simulink model "sim_assignment_drive"  (R2025b)
settings: Solver=VariableStepAuto  StartTime=0.0  StopTime=5*tau_tes  RelTol=1e-3
values from neighbouring files (symbols this model uses):
  conv = 3/Nav    (= 4.98173364331e-24)    [ass1_fuelcycle_cycle.m]    (also in ass1_steady_state.m)
  Efus_J = Efus*1.602e-13    (= 2.81952e-12)    [ass1_fuelcycle_cycle.m]    (also in ass1_steady_state.m)
  eta_tes = 0.9    [ass1_fuelcycle_cycle.m]    (also in ass1_steady_state.m)
  f_dir = 0.3    [ass1_fuelcycle_cycle.m]    (also in ass1_steady_state.m)
  I_inventory = I_inventory + 50    (= 1450)    [ass1_fuelcycle_cycle.m]    (also in ass1_steady_state.m)
  lambda = 1.83e-9    (= 1.83e-09)    [ass1_fuelcycle_cycle.m]    (also in ass1_steady_state.m)
  Pfus = 500e6    (= 500000000)    [ass1_fuelcycle_cycle.m]    (also in ass1_steady_state.m)
  pulse_width = t_pulse/t_period    (= 0.882352941176)    [ass1_fuelcycle_cycle.m]    (also in ass1_steady_state.m)
  t_period = t_pulse + t_dwell    (= 1020)    [ass1_fuelcycle_cycle.m]    (also in ass1_steady_state.m)
  tau_bb = 3600    [ass1_fuelcycle_cycle.m]    (also in ass1_steady_state.m)
  tau_cp = n_pumps*Mol_H/MolFR_H    [ass1_fuelcycle_cycle.m]    (also in ass1_steady_state.m)
  tau_hx = 3600    [ass1_fuelcycle_cycle.m]    (also in ass1_steady_state.m)
  tau_p = 6*3600    (= 21600)    [ass1_fuelcycle_cycle.m]    (also in ass1_steady_state.m)
  tau_tes = 24*3600    (= 86400)    [ass1_fuelcycle_cycle.m]    (also in ass1_steady_state.m)
  TBE = 0.01    [ass1_fuelcycle_cycle.m]    (also in ass1_steady_state.m)
settings Model: Creator=franc  LastModifiedBy=vairp

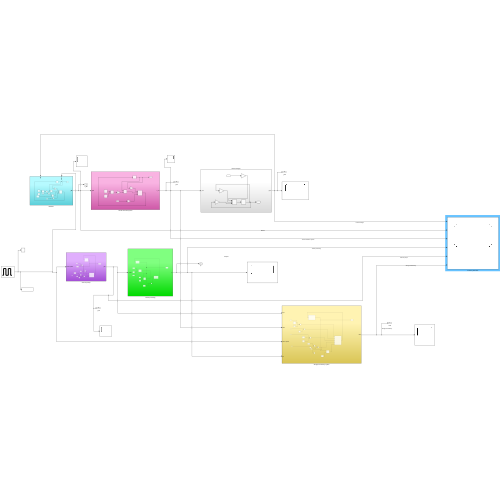
[thumbnail: Simulink's stored preview of the top-level diagram]
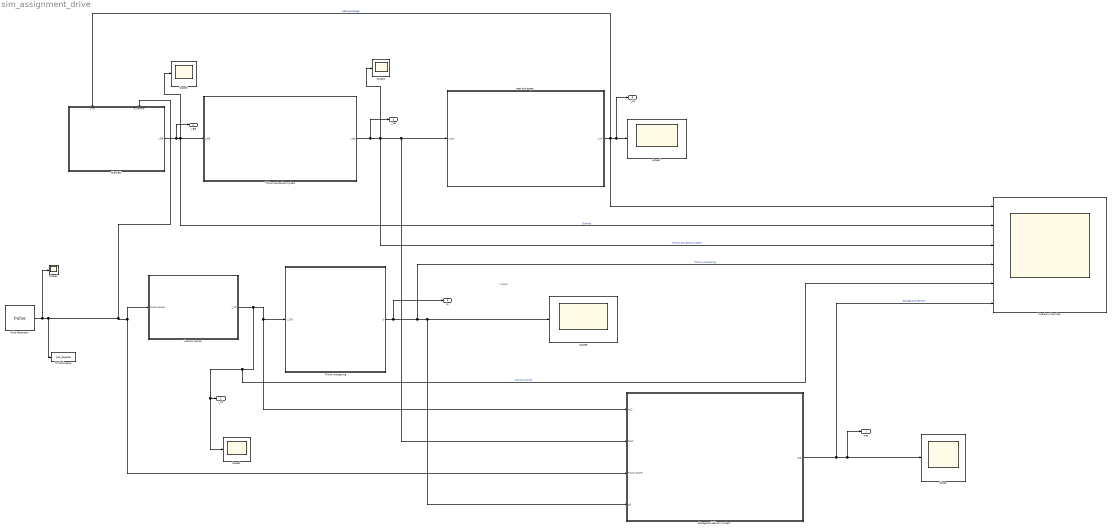
== system sim_assignment_drive ==
  note: scopew
  Blanket1 : Subsystem
      settings: PortSchema="{\"entries\":[{\"content\":{\"sides\":[{\"content\":{},\"type\":\"ConnectorPlacement.EquallySpacedRectSide\",\"uuid\":\"89bca18e-32ff-45a0-b030-61f554edbcca\"},{\"content\":{\"connectorIds\":[\"Out1\"],\"side\":\"RIGHT\"},\"type\":\"ConnectorPlacement.EquallySpacedRectSide\",\"uuid\":\"cf46e808-8a5d-458b-80f9-3800ce8b9836\"},{\"content\":{\"connectorIds\":[\"In1\",\"In2\"],\"side\":\"TOP\"},\"type\":\"ConnectorPlacement.EquallySpacedRectSide\",\"uuid\":\"39017523-1075-4513-926d-a7f0d16af0bc\"},{\"content\":{\"side\":\"BOTTOM\"},\"type\":\"ConnectorPlacement.EquallySpacedRectSide\",\"uuid\":\"04c0dc08-a93f-4928-be32-40ebfd4b2de5\"}]},\"type\":\"ConnectorPlacement.EquallySpacedConnector\",\"uuid\":\"6c4882b1-7a3e-4492-b971-e4bf86d91c33\"}],\"packageUris\":[\"http://schema.mathworks.com/mf0/Connector/R2020b\"],\"version\":\"1.0\"}"
  Heat exchanger : Subsystem
  Inventory Overview : Scope  NumInputPorts=6
      settings: ActiveDisplayYMinimum=-0.43034778362690795  ActiveDisplayYMaximum=3.8731300526421726  YLabel=Trtium inventory [g]  DataLoggingVariableName=ScopeData7
  Pulse Generator : DiscretePulseGenerator  PulseType=Time based  Amplitude=Pfus  Period=t_period  PulseWidth=pulse_width*100
  Scope{,1..5,7} (7 alike) : Scope
      Scope settings: ActiveDisplayYMinimum=35.349526834530543  ActiveDisplayYMaximum=54.275962480479521
      Scope1 settings: ActiveDisplayYMinimum=161.53440000057978  ActiveDisplayYMaximum=182.06300437811379
      Scope2 settings: ActiveDisplayYMinimum=-0.24605784431503164  ActiveDisplayYMaximum=3.8524924759412356  DataLoggingVariableName=ScopeData2
      Scope3 settings: ActiveDisplayYMinimum=-10.069495783527454  ActiveDisplayYMaximum=90.6254620517471  DataLoggingVariableName=ScopeData3
      Scope4 settings: ActiveDisplayYMinimum=-3.526352901457572E+7  ActiveDisplayYMaximum=5.0463497006759679E+8  DataLoggingVariableName=ScopeData4
      Scope5 settings: ActiveDisplayYMinimum=1163.0001078029038  ActiveDisplayYMaximum=1167.301162663447  DataLoggingVariableName=ScopeData5
      Scope7 settings: ActiveDisplayYMinimum=0.33167850023106693  ActiveDisplayYMaximum=0.33586626341534481  DataLoggingVariableName=ScopeData8
  Storage and delivery system : Subsystem
  To Workspace : ToWorkspace  VariableName=out_square  SaveFormat=Timeseries  SampleTime=-1
  Tritium extraction system : Subsystem
  Tritium processing : Subsystem
  Vacuum pumps : Subsystem
  Isds : Outport
  I_CP : Outport  Port=2
  Ip : Outport  Port=3
  I_BB : Outport  Port=4
  I_tes : Outport  Port=5
  I_HX : Outport  Port=6
  wires:
  Pulse Generator/1 -> Scope4/1, To Workspace/1, Storage and delivery system/3(Fusion power), Vacuum pumps/1(Fusion power), Blanket1/2(P_fusione)
  Vacuum pumps/1(I_CP) -> Inventory Overview/5, Scope1/1, I_CP/1, Storage and delivery system/1(Icp2), Tritium processing/1(I_CP2)  "Vacuum pumps"
  Heat exchanger/1(I_HX) -> I_HX/1, Scope7/1, Blanket1/1(I_HX), Inventory Overview/1  "Heat exchanger"
  Blanket1/1(I_BB) -> I_BB/1, Inventory Overview/2, Scope2/1, Tritium extraction system/1(I_BB)  "Blanket"
  Tritium extraction system/1(I_tes) -> I_tes/1, Inventory Overview/3, Scope3/1, Storage and delivery system/2(Ites2), Heat exchanger/1(I_tes)  "Tritium extraction system"
  Storage and delivery system/1(Isds) -> Inventory Overview/6, Isds/1, Scope/1  "Storage and delivery"
  Tritium processing/1(Ip) -> Ip/1, Inventory Overview/4, Storage and delivery system/4(Ip3), Scope5/1  "Tritium processing"

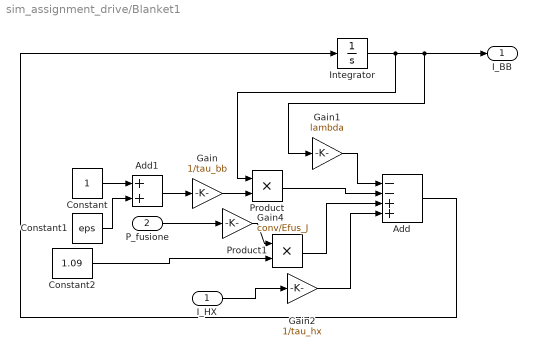
== system sim_assignment_drive/Blanket1 ==
  I_HX : Inport
  P_fusione : Inport  Port=2
  Add : Sum  Inputs=--++
  Add1 : Sum
  Constant : Constant
  Constant1 : Constant  Value=eps
  Constant2 : Constant  Value=1.09
  Gain : Gain  Gain=1/tau_bb
  Gain1 : Gain  Gain=lambda
  Gain2 : Gain  Gain=1/tau_hx
  Gain4 : Gain  Gain=conv/Efus_J
  Integrator : Integrator
  Product : Product
  Product1 : Product
  I_BB : Outport
  wires:
  Product1/1 -> Add/3
  Gain2/1 -> Add/4
  I_HX/1 -> Gain2/1
  Gain1/1 -> Add/1
  Product/1 -> Add/2
  Integrator/1 -> I_BB/1, Gain1/1, Product/1
  Gain/1 -> Product/2
  Add1/1 -> Gain/1
  Constant/1 -> Add1/1
  Constant1/1 -> Add1/2
  Add/1 -> Integrator/1
  Gain4/1 -> Product1/1
  Constant2/1 -> Product1/2
  P_fusione/1 -> Gain4/1

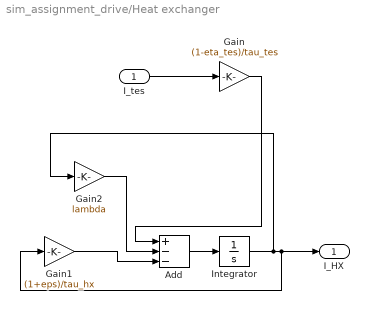
== system sim_assignment_drive/Heat exchanger ==
  I_tes : Inport
  Add : Sum  Inputs=+--
  Gain : Gain  Gain=(1-eta_tes)/tau_tes
  Gain1 : Gain  Gain=(1+eps)/tau_hx
  Gain2 : Gain  Gain=lambda
  Integrator : Integrator
  I_HX : Outport
  wires:
  I_tes/1 -> Gain/1
  Integrator/1 -> Gain2/1, Gain1/1, I_HX/1
  Gain/1 -> Add/1
  Gain1/1 -> Add/3
  Gain2/1 -> Add/2
  Add/1 -> Integrator/1

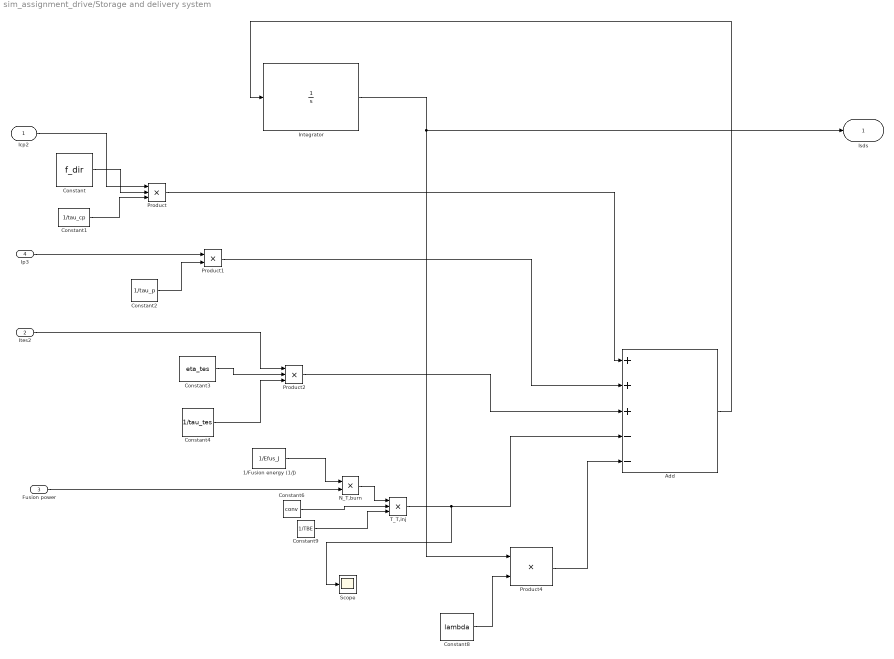
== system sim_assignment_drive/Storage and delivery system ==
  Icp2 : Inport
  Ites2 : Inport  Port=2
  Fusion power : Inport  Port=3
  Ip3 : Inport  Port=4
  1/Fusion energy (1/J) : Constant  Value=1/Efus_J
  Add : Sum  Inputs=+++--
  Constant : Constant  Value=f_dir
  Constant1 : Constant  Value=1/tau_cp
  Constant2 : Constant  Value=1/tau_p
  Constant3 : Constant  Value=eta_tes
  Constant4 : Constant  Value=1/tau_tes
  Constant6 : Constant  Value=conv
  Constant8 : Constant  Value=lambda
  Constant9 : Constant  Value=1/TBE
  Integrator : Integrator  InitialCondition=I_inventory
  N_T,burn : Product
  Product : Product  Inputs=3
  Product1 : Product
  Product2 : Product  Inputs=3
  Product4 : Product
  Scope : Scope
      settings: ActiveDisplayYMinimum=0.078343647913614214  ActiveDisplayYMaximum=0.0983436479136142  DataLoggingVariableName=ScopeData6
  T_T,inj : Product  Inputs=3
  Isds : Outport
  wires:
  Ip3/1 -> Product1/1
  Fusion power/1 -> N_T,burn/2
  Integrator/1 -> Isds/1, Product4/1
  1/Fusion energy (1/J)/1 -> N_T,burn/1
  N_T,burn/1 -> T_T,inj/1
  Constant/1 -> Product/2
  Ites2/1 -> Product2/1
  Constant6/1 -> T_T,inj/2
  Icp2/1 -> Product/1
  Add/1 -> Integrator/1
  Product/1 -> Add/1
  Constant1/1 -> Product/3
  Constant2/1 -> Product1/2
  Constant3/1 -> Product2/2
  Constant4/1 -> Product2/3
  T_T,inj/1 -> Scope/1, Add/4
  Product1/1 -> Add/2
  Constant8/1 -> Product4/2
  Product2/1 -> Add/3
  Constant9/1 -> T_T,inj/3
  Product4/1 -> Add/5

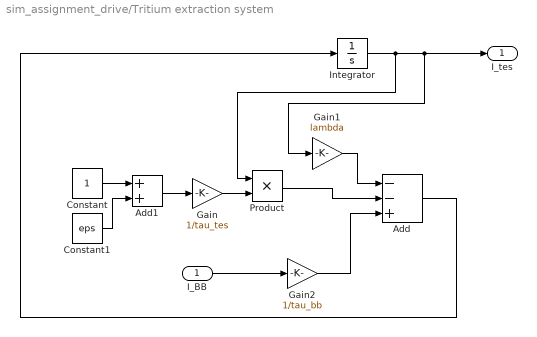
== system sim_assignment_drive/Tritium extraction system ==
  I_BB : Inport
  Add : Sum  Inputs=--+
  Add1 : Sum
  Constant : Constant
  Constant1 : Constant  Value=eps
  Gain : Gain  Gain=1/tau_tes
  Gain1 : Gain  Gain=lambda
  Gain2 : Gain  Gain=1/tau_bb
  Integrator : Integrator
  Product : Product
  I_tes : Outport
  wires:
  I_BB/1 -> Gain2/1
  Add/1 -> Integrator/1
  Gain2/1 -> Add/3
  Gain1/1 -> Add/1
  Product/1 -> Add/2
  Constant/1 -> Add1/1
  Constant1/1 -> Add1/2
  Add1/1 -> Gain/1
  Gain/1 -> Product/2
  Integrator/1 -> Product/1, Gain1/1, I_tes/1

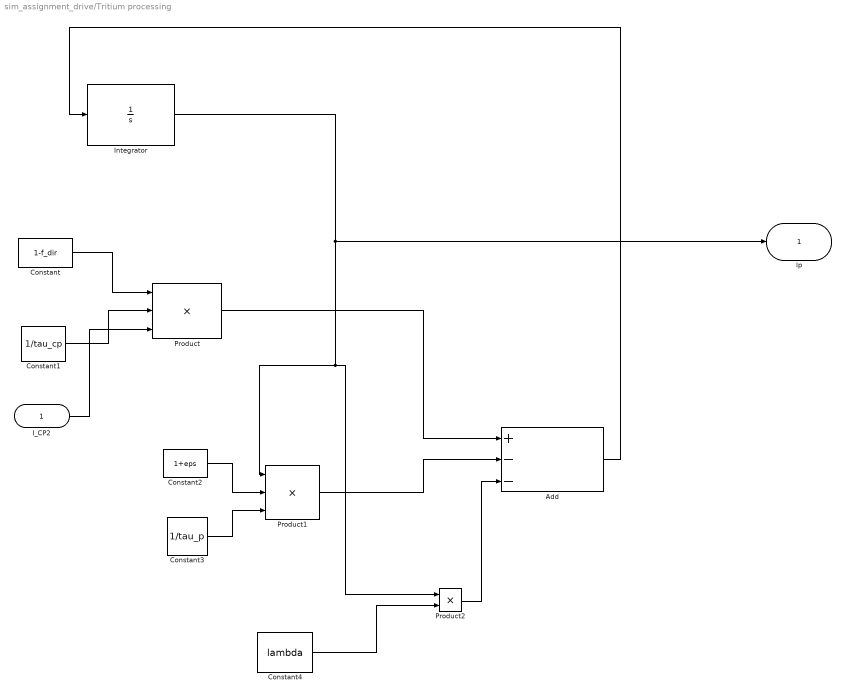
== system sim_assignment_drive/Tritium processing ==
  I_CP2 : Inport
  Add : Sum  Inputs=+--
  Constant : Constant  Value=1-f_dir
  Constant1 : Constant  Value=1/tau_cp
  Constant2 : Constant  Value=1+eps
  Constant3 : Constant  Value=1/tau_p
  Constant4 : Constant  Value=lambda
  Integrator : Integrator
  Product : Product  Inputs=3
  Product1 : Product  Inputs=3
  Product2 : Product
  Ip : Outport
  wires:
  Product1/1 -> Add/2
  Integrator/1 -> Ip/1, Product2/1, Product1/1
  Product2/1 -> Add/3
  Add/1 -> Integrator/1
  Constant4/1 -> Product2/2
  I_CP2/1 -> Product/3
  Constant2/1 -> Product1/2
  Constant/1 -> Product/1
  Constant1/1 -> Product/2
  Constant3/1 -> Product1/3
  Product/1 -> Add/1

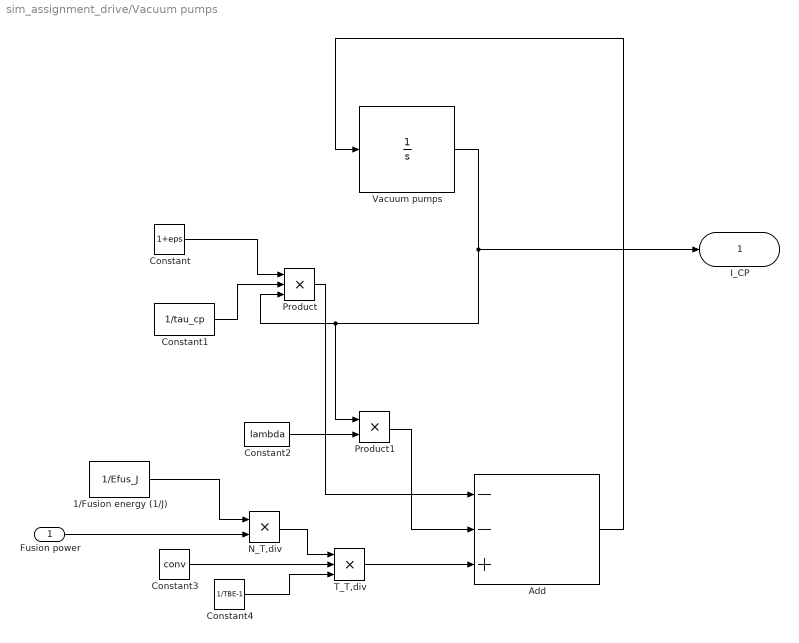
== system sim_assignment_drive/Vacuum pumps ==
  Fusion power : Inport
  1/Fusion energy (1/J) : Constant  Value=1/Efus_J
  Add : Sum  Inputs=--+
  Constant : Constant  Value=1+eps
  Constant1 : Constant  Value=1/tau_cp
  Constant2 : Constant  Value=lambda
  Constant3 : Constant  Value=conv
  Constant4 : Constant  Value=1/TBE-1
  N_T,div : Product
  Product : Product  Inputs=3
  Product1 : Product
  T_T,div : Product  Inputs=3
  Vacuum pumps : Integrator
  I_CP : Outport
  wires:
  Product1/1 -> Add/2
  Add/1 -> Vacuum pumps/1
  Vacuum pumps/1 -> I_CP/1, Product1/1, Product/3
  N_T,div/1 -> T_T,div/1
  Constant2/1 -> Product1/2
  Fusion power/1 -> N_T,div/2
  Constant/1 -> Product/1
  Constant1/1 -> Product/2
  Product/1 -> Add/1
  1/Fusion energy (1/J)/1 -> N_T,div/1
  Constant3/1 -> T_T,div/2
  T_T,div/1 -> Add/3
  Constant4/1 -> T_T,div/3
